simulink model "sfbuilder_stats"  (Simulink 7.6)
settings: Solver=ode5  StartTime=0.0  StopTime=500  RelTol=1e-3
settings Model: Creator=The MathWorks Inc.  ExtModeAutoUpdateStatusClock=off
settings DataIOCC: SignalLoggingName=sigsOut
settings OptimizationCC: InlineInvariantSignals=on  InitFltsAndDblsToZero=on  BufferReusableBoundary=off
settings DebuggingCC: SaveWithParameterizedLinksMsg=none  SignalResolutionControl=TryResolveAllWithWarning  SolverPrmCheckMsg=none  MultiTaskDSMMsg=warning  MultiTaskCondExecSysMsg=none
settings HardwareCC: TargetUnknown=on
settings RTWCC: IncludeERTFirstTime=on
settings GRTTargetCC: TargetFcnLib=ansi_tfl_tmw.mat

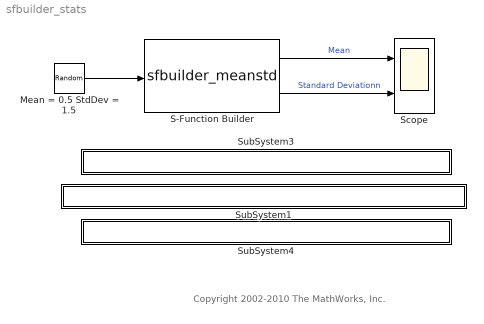
== system sfbuilder_stats ==
  note: Copyright 2002-2010 The MathWorks, Inc.
  Mean = 0.5 StdDev = 1.5 : RandomNumber  Mean=0.5  Variance=2.25  SampleTime=0.1
  S-Function Builder : S-Function  FunctionName=sfbuilder_meanstd  SFunctionModules=sfbuilder_meanstd_wrapper  WizardData=DataTag0  EnableBusSupport=off  mask(S-Function Builder){}
      mask init:
      | val = [[.9  0.75 0.75 1 1 .9 .9 1]',[1 1 0.75 0.75 .9 .9 1 .9]'];try , sys = get_param(gcb,'SfunBuilderFcnName');if isempty(sys), sys = get_param(gcb,'FunctionName'); end,catch, sys = get_param(gcb,'FunctionName'); end
      settings: CopyFcn=set_param(gcb,'LinkStatus','none')  OpenFcn=sfunctionwizard(gcbh)
      mask Display:
      | plot(val(:,1),val(:,2))
      | disp(sys)
      | port_label('input',1,'sig')
      | port_label('output',1,'Mean')
      | port_label('output',2,'stDeviation')
  Scope : Scope  NumInputPorts=2
      settings: TimeRange=500  YMin=0~0  YMax=2.5~2  SaveName=ScopeData2
  SubSystem1 : Subsystem  mask{filename=sfbuilder_meanstd_wrapper.c}
      mask init:
      | x=sfundemo_maskdisp;
      settings: AttributesFormatString=\n  OpenFcn=sfundemo_openfcn
      mask Display: disp(x);
  SubSystem3 : Subsystem  mask{filename=sfbuilder_meanstd.c}
      mask init:
      | x=sfundemo_maskdisp;
      settings: AttributesFormatString=\n  OpenFcn=sfundemo_openfcn
      mask Display: disp(x);
  SubSystem4 : Subsystem  mask{filename=sfbuilder_meanstd.tlc}
      mask init:
      | x=sfundemo_maskdisp;
      settings: AttributesFormatString=\n  OpenFcn=sfundemo_openfcn
      mask Display: disp(x);
  wires:
  Mean = 0.5 StdDev = 1.5/1 -> S-Function Builder/1
  S-Function Builder/1 -> Scope/1  "Mean"
  S-Function Builder/2 -> Scope/2  "Standard Deviationn"

== system sfbuilder_stats/SubSystem1 ==

== system sfbuilder_stats/SubSystem3 ==

== system sfbuilder_stats/SubSystem4 ==
